simulink model "tqdtqr_rebuild_V3"  (R2021b)
settings: Solver=VariableStepAuto  StartTime=0.0  StopTime=10.0  RelTol=1e-3
undefined symbols (not defined in the file): ATQD_AfterTqMinGain_X_Deg, ATQD_APSCreepBaseTqD_X_kph, ATQD_APSCreepBaseTqD_Y_Deg, ATQD_APSCreepBaseTqR_X_kph, ATQD_APSCreepBaseTqR_Y_Deg, ATQD_APSCreepIterm_X_kph, ATQD_APSCreepIterm_Y_kph, ATQD_APSCreepPterm_X_kph, ATQD_APSCreepPterm_Y_kph, ATQD_APSDecReq_X_kph, ATQD_APSDecReq_Y_mps2, ATQD_APSDecReqCMD_X_kph, ATQD_APSDecReqTs_X_pct, ATQD_APSDecTimeGain_X_Deg, ATQD_APSDecTimeGain_Y_s, ATQD_APSReqLowSpd_X_Deg, ATQD_AutoHoldReleaseBPS_X_Deg, ATQD_AWDLoadTrqnsGain_X_kg, ATQD_AWDLoadTrqnsGain_Y_pct, ATQD_BOSEnBPSPosn_X_kph, ATQD_BOSMap_X_rpm, ATQD_BOSMap_Y_pct, ATQD_CreepBaseTqD_X_kph, ATQD_CreepBaseTqD_Y_Deg, ATQD_CreepBaseTqR_X_kph, ATQD_CreepBaseTqR_Y_Deg, ATQD_CreepBPSDisPosn_X_Deg, ATQD_CreepBPSDisPosnR_X_Deg, ATQD_CreepBPSEnPosn_X_Deg, ATQD_CreepBPSEnPosnR_X_Deg, ATQD_CreepDeltaTq_X_kph, ATQD_CreepIterm_X_kph, ATQD_CreepIterm_Y_kph, ATQD_CreepItermMaxLimit_X_pct, ATQD_CreepPreloadTime_X_kph, ATQD_CreepPreloadTq_X_kph, ATQD_CreepPreloadTq_Y_s, ATQD_CreepProtTq_X_Deg, ATQD_CreepPterm_X_kph, ATQD_CreepPterm_Y_kph, ATQD_CreepRrTqSpRat_X_rpm, ATQD_CreepRrTqSpRat_Y_Nm, ATQD_CreepTargetSpdD_X_pct, ATQD_CreepTargetSpdR_X_pct, ATQD_CreepUpLimitTq_X_rpm, ATQD_DecIneOPDHoldEnDelay_X_Deg, ATQD_DecIneOPDHoldEnDelay_Y_bar, ATQD_ECOTqMapD_X_rpm, ATQD_ECOTqMapD_Y_pct, ATQD_EMTqMapD_X_rpm, ATQD_EMTqMapD_Y_pct, ATQD_EOPDTqMapDCon_X_rpm, ATQD_EOPDTqMapDCon_Y_Deg, ATQD_EstInitVehWeight_X_c, ATQD_FAfterTqCMDGain_X_rpm, ATQD_FAfterTqCMDGain_Y_pct, ATQD_ForceLowSpd_X_Deg, ATQD_ForcePLimitSpd_X_Deg, ATQD_FrLossMAPLowV_X_rpm, ATQD_FrLossMAPLowV_Y_Nm ... (+949)
libraries: simulink x235, hcu_lib x208, tqr x63, tqd x6
(part 8 of 37)

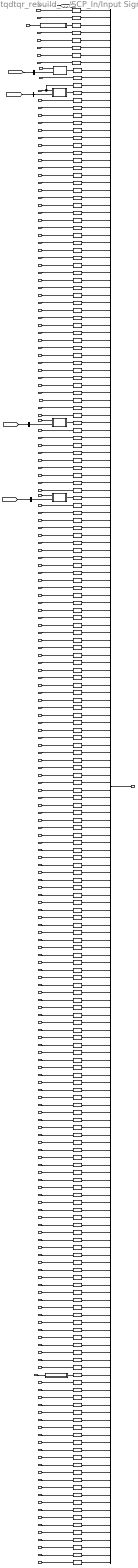
== system tqdtqr_rebuild_V3/SCP_In/Input Signal ==
  BInInvalid_outputs : Inport
  task_time_s : Inport  Port=2
  VDHP_ActAPSPosn_pct : Inport  Port=3
  VDHP_LowIdleAccPedal_flg : Inport  Port=4
  VPMM_PowerSta_enum : Inport  Port=5
  VPMM_DrivetrainSelect_enum : Inport  Port=6
  VPMM_SysPowerMode_enum : Inport  Port=7
  VPMM_DrSeatSta_enum : Inport  Port=8
  VINP_VehSpeed_kph : Inport  Port=9
  VINP_BrkSwSta_flg : Inport  Port=10
  VINP_BrkSwV_flg : Inport  Port=11
  VINP_BrkPedalPos_pct : Inport  Port=12
  VINP_BrkPedalPosSta_flg : Inport  Port=13
  VINP_FrPTCSActive_flg : Inport  Port=14
  VINP_RrPTCSActive_flg : Inport  Port=15
  VINP_FrntAxlTrqReqDrv_Nm : Inport  Port=16
  VINP_RearAxlTrqReqDrv_Nm : Inport  Port=17
  VINP_FrRBCActive_flg : Inport  Port=18
  VINP_RrRBCActive_flg : Inport  Port=19
  VINP_FrntAxlTrqReqBrk_Nm : Inport  Port=20
  VINP_RearAxlTrqReqBrk_Nm : Inport  Port=21
  VINP_CrashOutputSts_enum : Inport  Port=22
  VINP_LongAccel_Gps : Inport  Port=23
  VINP_EPBCarWashMode_flg : Inport  Port=24
  VINP_EPBErrSta_enum : Inport  Port=25
  VINP_EPBSta_enum : Inport  Port=26
  VINP_DOASta_flg : Inport  Port=27
  VINP_GRADE_Deg : Inport  Port=28
  VINP_HSAActive_flg : Inport  Port=29
  VINP_DriverSeatBeltCmd_flg : Inport  Port=30
  VINP_AVHActive_flg : Inport  Port=31
  VINP_PsngrSeatBeltCmd_flg : Inport  Port=32
  VINP_RDriverSeatBeltCmd_flg : Inport  Port=33
  VINP_RCenterSeatBeltCmd_flg : Inport  Port=34
  VINP_RPsngrSeatBeltCmd_flg : Inport  Port=35
  VINP_YawRate_degps : Inport  Port=36
  VINP_SASAngle_Deg : Inport  Port=37
  VINP_ESCActive_flg : Inport  Port=38
  VINP_ABSActive_flg : Inport  Port=39
  VINP_LFRawWhlSpeed_kph : Inport  Port=40
  VINP_LRRawWhlSpeed_kph : Inport  Port=41
  VINP_RFRawWhlSpeed_kph : Inport  Port=42
  VINP_RRRawWhlSpeed_kph : Inport  Port=43
  VINP_ESCOFFStatus_enum : Inport  Port=44
  VINP_MCPressure_bar : Inport  Port=45
  VINP_IVIPWModeReq_enum : Inport  Port=46
  VINP_IVICreepSWReq_flg : Inport  Port=47
  VINP_RollModeSWCmd_enum : Inport  Port=48
  VINP_IVIPwrLockSW_enum : Inport  Port=49
  VINP_IVIISAOffsetSpd_enum : Inport  Port=50
  VINP_Distanceunit_flg : Inport  Port=51
  VINP_SmartEcoModeSW_flg : Inport  Port=52
  VINP_IVISnowModeCmd_flg : Inport  Port=53
  VINP_IVIACCAdaptiveSta_flg : Inport  Port=54
  VINP_IVITrailerModeSWSta_flg : Inport  Port=55
  VINP_ShifterHandleCmd_enum : Inport  Port=56
  VINP_HVBPwrAvailDchrg_kW : Inport  Port=57
  VINP_HVBPwrAvailChrg_kW : Inport  Port=58
  VINP_HVBattErr_flg : Inport  Port=59
  VINP_DCDCFaultSta_enum : Inport  Port=60
  VINP_ChrgPlugSta_enum : Inport  Port=61
  VINP_HVBattSOC_pct : Inport  Port=62
  VINP_HVBattSOCDis_pct : Inport  Port=63
  VINP_HVBMTempMax_C : Inport  Port=64
  VINP_HVBMTempMin_C : Inport  Port=65
  VINP_ShifterFailsta_enum : Inport  Port=66
  VINP_CANMsgValidMCUNR1_flg : Inport  Port=67
  VINP_FrEDURotateDirctionNidec_enum : Inport  Port=68
  VINP_FrEDURotateDirction_enum : Inport  Port=69
  VINP_RrEDURotateDirctionNidec_enum : Inport  Port=70
  VINP_RrEDURotateDirction_enum : Inport  Port=71
  VINP_FrTMSpdNidec_rpm : Inport  Port=72
  VINP_FrTMSpd_rpm : Inport  Port=73
  VINP_RrTMSpdNidec_rpm : Inport  Port=74
  VINP_RrTMSpd_rpm : Inport  Port=75
  VINP_FrRegenAvailTqNidec_Nm : Inport  Port=76
  VINP_FrRegenAvailTq_Nm : Inport  Port=77
  VINP_RrRegenAvailTqNidec_Nm : Inport  Port=78
  VINP_RrRegenAvailTq_Nm : Inport  Port=79
  VINP_FrEDURealTMTqNidec_Nm : Inport  Port=80
  VINP_FrEDURealTMTq_Nm : Inport  Port=81
  VINP_RrEDURealTMTqNidec_Nm : Inport  Port=82
  VINP_RrEDURealTMTq_Nm : Inport  Port=83
  VINP_FrMotorAvailTqNidec_Nm : Inport  Port=84
  VINP_FrMotorAvailTq_Nm : Inport  Port=85
  VINP_RrMotorAvailTqNidec_Nm : Inport  Port=86
  VINP_RrMotorAvailTq_Nm : Inport  Port=87
  VINP_MCUWarnFNidec_enum : Inport  Port=88
  VINP_MCUWarnF_enum : Inport  Port=89
  VINP_MCUWarnRNidec_enum : Inport  Port=90
  VINP_MCUWarnR_enum : Inport  Port=91
  VINP_FrMCUDCBusVoltNidec_V : Inport  Port=92
  VINP_FrMCUDCBusVolt_V : Inport  Port=93
  VINP_RrMCUDCBusVoltNidec_V : Inport  Port=94
  VINP_RrMCUDCBusVolt_V : Inport  Port=95
  VINP_FrMCUTempNidec_C : Inport  Port=96
  VINP_FrMCUTemp_C : Inport  Port=97
  VINP_FrTMTempNidec_C : Inport  Port=98
  VINP_FrTMTemp_C : Inport  Port=99
  VINP_RrMCUTempNidec_C : Inport  Port=100
  VINP_RrMCUTemp_C : Inport  Port=101
  VINP_RrTMTempNidec_C : Inport  Port=102
  VINP_RrTMTemp_C : Inport  Port=103
  VINP_SWCResUpSta_flg : Inport  Port=104
  VINP_SWCSetdownSta_flg : Inport  Port=105
  VINP_SWCACCSta_flg : Inport  Port=106
  VINP_SWCCANCELSta_flg : Inport  Port=107
  VINP_SWC2LScrollUpSta_flg : Inport  Port=108
  VINP_SWC2LScrollDownSta_flg : Inport  Port=109
  VINP_SWC2LScrollPressSta_flg : Inport  Port=110
  VINP_SWC2LADASSta_flg : Inport  Port=111
  VINP_SWC2RScrollPressSta_flg : Inport  Port=112
  VINP_SWC2RScrollUpSta_flg : Inport  Port=113
  VINP_SWC2RScrollDownSta_flg : Inport  Port=114
  VINP_SWC2LDriveModeSta_flg : Inport  Port=115
  VINP_SWC2RRightSta_flg : Inport  Port=116
  VINP_SWC2RLeftSta_flg : Inport  Port=117
  VINP_SWCRegenUp_flg : Inport  Port=118
  VINP_SWC2RCustomizeSta_flg : Inport  Port=119
  VINP_SWC2LRegenUpSta_flg : Inport  Port=120
  VINP_SWC2RRegenDownSta_flg : Inport  Port=121
  VINP_SWCRegenDown_flg : Inport  Port=122
  VVMC_ADASForceIdle_flg : Inport  Port=123
  VVMC_ACCRequiredAccel_mps2 : Inport  Port=124
  VVMC_ACCVehHoldReq_flg : Inport  Port=125
  VVMC_ADASActive_flg : Inport  Port=126
  VVMC_ADASWhlTqReq_Nm : Inport  Port=127
  VVMC_CruzActive_flg : Inport  Port=128
  VVMC_CruzWhlTqReq_Nm : Inport  Port=129
  VVMC_MSAActive_flg : Inport  Port=130
  VVMC_MSAWhlTqReq_Nm : Inport  Port=131
  VVMC_APSActive_flg : Inport  Port=132
  VVMC_APSSpeedCMD_kph : Inport  Port=133
  VVMC_APSShiftPosnReq_enum : Inport  Port=134
  VVMC_ACCPedalOvrd_flg : Inport  Port=135
  VVMC_LongAcc_Gps : Inport  Port=136
  VVMC_ActMaxSlideRate_pct : Inport  Port=137
  VVMC_EstSlope_Deg : Inport  Port=138
  VVMC_APSReq_enum : Inport  Port=139
  VVMC_RWDRDCActive_enum : Inport  Port=140
  VVMC_ActLRSlideRate_pct : Inport  Port=141
  VVMC_ActRRSlideRate_pct : Inport  Port=142
  VVMC_ActStESCYaw_Dps : Inport  Port=143
  VVMC_CCCtrlSta_enum : Inport  Port=144
  VVMC_MSACtrlSta_enum : Inport  Port=145
  VVMC_LVDAACCStatusInformation_flg : Inport  Port=146
  VVMC_ACCObjDist_m : Inport  Port=147
  VVMC_MeterIndSpeed_raw32 : Inport  Port=148
  VVMC_RearTqRatio_rat : Inport  Port=149
  VVMC_CalibratedGyroY_Dps : Inport  Port=150
  VVMC_CAASActive_flg : Inport  Port=151
  VVMC_SetACCDisableAPS_flg : Inport  Port=152
  VVMC_CCPedalOvrd_flg : Inport  Port=153
  VVMC_MSAWhlTqActive_flg : Inport  Port=154
  VINP_BrakeSWGPIO_flg : Inport  Port=155
  VINP_CrashSignalGPIO_flg : Inport  Port=156
  VINP_DrDoorSW_flg : Inport  Port=157
  VINP_SeatSW_flg : Inport  Port=158
  VINP_HoodSW_flg : Inport  Port=159
  VINP_TailgateSW_flg : Inport  Port=160
  VINP_PsDoorSW_flg : Inport  Port=161
  VINP_RRDoorSW_flg : Inport  Port=162
  VINP_RLDoorSW_flg : Inport  Port=163
  VBCM_BrakeLamp_flg : Inport  Port=164
  VBCM_UserNow_enum : Inport  Port=165
  VINP_ADASISASta_enum : Inport  Port=166
  VINP_ADASVehSpdLim_enum : Inport  Port=167
  VINP_ADASACCSta_enum : Inport  Port=168
  VINP_ADASSLIFSpdLim_enum : Inport  Port=169
  VINP_ADASAEBSta_enum : Inport  Port=170
  VINP_ACCVehHoldReq_flg : Inport  Port=171
  VINP_FlashRegenMode_enum : Inport  Port=172
  VINP_VehicleType_enum : Inport  Port=173
  VINP_SWCType_enum : Inport  Port=174
  VINP_CAASSta_enum : Inport  Port=175
  VINP_APSStaSystem_enum : Inport  Port=176
  VDDM_VCURAPSErrLv2_flg : Inport  Port=177
  VDDM_VCURAPSErrLv3_flg : Inport  Port=178
  VDDM_EPBSigErrCFS_flg : Inport  Port=179
  VDDM_EPB1Err_flg : Inport  Port=180
  VDDM_ESC1Err_flg : Inport  Port=181
  VDDM_ESC5Err_flg : Inport  Port=182
  VDDM_LimpHomeAct_flg : Inport  Port=183
  VDDM_VehMalfunLevel_enum : Inport  Port=184
  VDDM_Shifter1Err_flg : Inport  Port=185
  VDDM_ShifterSigErrCFS_flg : Inport  Port=186
  VDDM_MCUF1Err_flg : Inport  Port=187
  VDDM_MCUR1Err_flg : Inport  Port=188
  VDDM_RegenErrCFS_flg : Inport  Port=189
  VDDM_4D2CErr_flg : Inport  Port=190
  VINP_PBWMotorPos_enum : Inport  Port=191
  VBCM_RegenModeUserSetting_enum : Inport  Port=192
  VINP_IVIEscapeModeCmd_flg : Inport  Port=193
  VINP_DIDExhibitMode_enum : Inport  Port=194
  VINP_DIDGetDynoMode_flg : Inport  Port=195
  VINP_CAN1BusOff_flg : Inport  Port=196
  VINP_CAN1BusError_flg : Inport  Port=197
  VINP_CAN2BusOff_flg : Inport  Port=198
  VINP_CAN2BusError_flg : Inport  Port=199
  VINP_DIDNVHPedalLim_flg : Inport  Port=200
  VINP_SCPSystemMode_enum : Inport  Port=201
  VDDM_EPB1NoComCFS_flg : Inport  Port=202
  VDDM_EPB1RCErrCFS_flg : Inport  Port=203
  VDDM_EPB1CSErrCFS_flg : Inport  Port=204
  VBCM_CTDCtrl_enum : Inport  Port=205
  VINP_FlashCrashDetd_flg : Inport  Port=206
  VINP_FlashCrashUnlockReq_flg : Inport  Port=207
  VBCM_CrashUnlkSuccess_flg : Inport  Port=208
  BrkPedalPos : Subsystem
  BrkSwSta : Subsystem
  Bus Creator : BusCreator  Inputs=208
  Bus Selector1 : BusSelector  OutputSignals=VTQD_ShifterHandleCmdInV_flg
  Bus Selector2 : BusSelector  OutputSignals=VTQD_ShifterFailstaInV_flg
  Bus Selector3 : BusSelector  OutputSignals=VINP_BrkSwStaSWInV_flg
  Bus Selector4 : BusSelector  OutputSignals=VINP_BrkPedalPosStaInV_flg
  Data Type Conversion{,1,6,9,13..14,17..18,20,25,33..34,37..40,53..54,58..61,68..83,88..99,120,123,125,127,129,132..134,137..139,143..146,191,203} (67 alike) : DataTypeConversion  OutDataTypeStr=single
  Data Type Conversion{2,7..8,10..12,15..16,21,24,26..32,35..36,43,47..51,55,63,100..119,121..122,124,126,128,131,142,147..158,170..176,178..183,185..190,192..196,199..201,205..207} (96 alike) : DataTypeConversion  OutDataTypeStr=boolean
  Data Type Conversion{3..5,19,22..23,41..42,44..46,52,56..57,62,64..67,84..87,130,135..136,140..141,159..169,177,184,197..198,202,204} (45 alike) : DataTypeConversion  OutDataTypeStr=uint8
  ShifterFailsta : Subsystem
  ShifterHandleCmd : Subsystem
  VDDM_LimpHomeAct_flg_ovrd : Subsystem
  VDHP_LowIdleAccPedal_flg_ovrd : Subsystem
  BSCPIn_outputs : Outport
  wires:
  Data Type Conversion177/1 -> Bus Creator/184  "VDDM_VehMalfunLevel_enum"
  Data Type Conversion184/1 -> Bus Creator/191  "VINP_PBWMotorPos_enum"
  VINP_EPBCarWashMode_flg/1 -> Data Type Conversion21/1
  Data Type Conversion107/1 -> Bus Creator/111  "VINP_SWC2LADASSta_flg"
  Data Type Conversion45/1 -> Bus Creator/49  "VINP_IVIPwrLockSW_enum"
  Data Type Conversion173/1 -> Bus Creator/180  "VDDM_EPB1Err_flg"
  VINP_RrMCUTemp_C/1 -> Data Type Conversion97/1
  VINP_ADASSLIFSpdLim_enum/1 -> Data Type Conversion163/1
  Data Type Conversion172/1 -> Bus Creator/179  "VDDM_EPBSigErrCFS_flg"
  Data Type Conversion179/1 -> Bus Creator/186  "VDDM_ShifterSigErrCFS_flg"
  Data Type Conversion148/1 -> Bus Creator/152  "VVMC_SetACCDisableAPS_flg"
  Data Type Conversion134/1 -> Bus Creator/138  "VVMC_EstSlope_Deg"
  Data Type Conversion108/1 -> Bus Creator/112  "VINP_SWC2RScrollPressSta_flg"
  Data Type Conversion127/1 -> Bus Creator/131  "VVMC_MSAWhlTqReq_Nm"
  VINP_CrashSignalGPIO_flg/1 -> Data Type Conversion150/1
  VINP_IVISnowModeCmd_flg/1 -> Data Type Conversion49/1
  VINP_IVIEscapeModeCmd_flg/1 -> Data Type Conversion186/1
  Data Type Conversion139/1 -> Bus Creator/143  "VVMC_ActStESCYaw_Dps"
  Data Type Conversion105/1 -> Bus Creator/109  "VINP_SWC2LScrollDownSta_flg"
  Data Type Conversion47/1 -> Bus Creator/51  "VINP_Distanceunit_flg"
  Data Type Conversion118/1 -> Bus Creator/122  "VINP_SWCRegenDown_flg"
  VINP_DCDCFaultSta_enum/1 -> Data Type Conversion56/1
  VINP_ADASISASta_enum/1 -> Data Type Conversion160/1
  VDDM_Shifter1Err_flg/1 -> Data Type Conversion178/1
  Data Type Conversion71/1 -> Bus Creator/75  "VINP_RrTMSpd_rpm"
  Data Type Conversion175/1 -> Bus Creator/182  "VDDM_ESC5Err_flg"
  Data Type Conversion171/1 -> Bus Creator/178  "VDDM_VCURAPSErrLv3_flg"
  Data Type Conversion32/1 -> Bus Creator/35  "VINP_RPsngrSeatBeltCmd_flg"
  Data Type Conversion140/1 -> Bus Creator/144  "VVMC_CCCtrlSta_enum"
  Data Type Conversion/1 -> Bus Creator/1  "task_time_s"
  Data Type Conversion131/1 -> Bus Creator/135  "VVMC_ACCPedalOvrd_flg"
  VINP_RrEDURealTMTqNidec_Nm/1 -> Data Type Conversion78/1
  Data Type Conversion89/1 -> Bus Creator/93  "VINP_FrMCUDCBusVolt_V"
  VDDM_ShifterSigErrCFS_flg/1 -> Data Type Conversion179/1
  Data Type Conversion126/1 -> Bus Creator/130  "VVMC_MSAActive_flg"
  VINP_RPsngrSeatBeltCmd_flg/1 -> Data Type Conversion32/1
  Data Type Conversion24/1 -> Bus Creator/27  "VINP_DOASta_flg"
  VINP_SWC2LScrollDownSta_flg/1 -> Data Type Conversion105/1
  Data Type Conversion174/1 -> Bus Creator/181  "VDDM_ESC1Err_flg"
  VDDM_EPB1Err_flg/1 -> Data Type Conversion173/1
  VINP_CAASSta_enum/1 -> Data Type Conversion168/1
  Data Type Conversion38/1 -> Bus Creator/41  "VINP_LRRawWhlSpeed_kph"
  Data Type Conversion75/1 -> Bus Creator/79  "VINP_RrRegenAvailTq_Nm"
  VVMC_ActLRSlideRate_pct/1 -> Data Type Conversion137/1
  VINP_RDriverSeatBeltCmd_flg/1 -> Data Type Conversion30/1
  Data Type Conversion116/1 -> Bus Creator/120  "VINP_SWC2LRegenUpSta_flg"
  Data Type Conversion11/1 -> Bus Creator/14  "VINP_FrPTCSActive_flg"
  VINP_ADASAEBSta_enum/1 -> Data Type Conversion164/1
  Data Type Conversion176/1 -> Bus Creator/183  "VTQD_LimpHomeAct_flg"
  VVMC_ActRRSlideRate_pct/1 -> Data Type Conversion138/1
  Data Type Conversion94/1 -> Bus Creator/98  "VINP_FrTMTempNidec_C"
  Data Type Conversion178/1 -> Bus Creator/185  "VDDM_Shifter1Err_flg"
  Data Type Conversion121/1 -> Bus Creator/125  "VVMC_ACCVehHoldReq_flg"
  Data Type Conversion138/1 -> Bus Creator/142  "VVMC_ActRRSlideRate_pct"
  VDDM_MCUR1Err_flg/1 -> Data Type Conversion181/1
  Data Type Conversion76/1 -> Bus Creator/80  "VINP_FrEDURealTMTqNidec_Nm"
  Data Type Conversion182/1 -> Bus Creator/189  "VDDM_RegenErrCFS_flg"
  Data Type Conversion103/1 -> Bus Creator/107  "VINP_SWCCANCELSta_flg"
  Data Type Conversion183/1 -> Bus Creator/190  "VDDM_4D2CErr_flg"
  Data Type Conversion157/1 -> Bus Creator/163  "VINP_RLDoorSW_flg"
  Data Type Conversion98/1 -> Bus Creator/102  "VINP_RrTMTempNidec_C"
  Data Type Conversion185/1 -> Bus Creator/192  "VBCM_RegenModeUserSetting_enum"
  VVMC_SetACCDisableAPS_flg/1 -> Data Type Conversion148/1
  VINP_LFRawWhlSpeed_kph/1 -> Data Type Conversion37/1
  Data Type Conversion21/1 -> Bus Creator/24  "VINP_EPBCarWashMode_flg"
  Data Type Conversion99/1 -> Bus Creator/103  "VINP_RrTMTemp_C"
  VINP_HVBMTempMin_C/1 -> Data Type Conversion61/1
  Data Type Conversion119/1 -> Bus Creator/123  "VVMC_ADASForceIdle_flg"
  Data Type Conversion18/1 -> Bus Creator/21  "VINP_RearAxlTrqReqBrk_Nm"
  VVMC_RearTqRatio_rat/1 -> Data Type Conversion145/1
  Data Type Conversion50/1 -> Bus Creator/54  "VINP_IVIACCAdaptiveSta_flg"
  Data Type Conversion55/1 -> Bus Creator/59  "VINP_HVBattErr_flg"
  VINP_DriverSeatBeltCmd_flg/1 -> Data Type Conversion27/1
  VINP_HVBPwrAvailChrg_kW/1 -> Data Type Conversion54/1
  VVMC_ActStESCYaw_Dps/1 -> Data Type Conversion139/1
  Data Type Conversion129/1 -> Bus Creator/133  "VVMC_APSSpeedCMD_kph"
  VINP_ESCActive_flg/1 -> Data Type Conversion35/1
  Data Type Conversion180/1 -> Bus Creator/187  "VDDM_MCUF1Err_flg"
  Data Type Conversion104/1 -> Bus Creator/108  "VINP_SWC2LScrollUpSta_flg"
  Bus Creator/1 -> BSCPIn_outputs/1  "BSCPIn_outputs"
  Data Type Conversion73/1 -> Bus Creator/77  "VINP_FrRegenAvailTq_Nm"
  Data Type Conversion4/1 -> Bus Creator/5  "VPMM_DrivetrainSelect_enum"
  Data Type Conversion97/1 -> Bus Creator/101  "VINP_RrMCUTemp_C"
  Data Type Conversion26/1 -> Bus Creator/29  "VINP_HSAActive_flg"
  Data Type Conversion181/1 -> Bus Creator/188  "VDDM_MCUR1Err_flg"
  Data Type Conversion46/1 -> Bus Creator/50  "VINP_IVIISAOffsetSpd_enum"
  Data Type Conversion186/1 -> Bus Creator/193  "VINP_IVIEscapeModeCmd_flg"
  Data Type Conversion113/1 -> Bus Creator/117  "VINP_SWC2RLeftSta_flg"
  Data Type Conversion96/1 -> Bus Creator/100  "VINP_RrMCUTempNidec_C"
  Data Type Conversion60/1 -> Bus Creator/64  "VINP_HVBMTempMax_C"
  VINP_FrntAxlTrqReqBrk_Nm/1 -> Data Type Conversion17/1
  Data Type Conversion90/1 -> Bus Creator/94  "VINP_RrMCUDCBusVoltNidec_V"
  VINP_FrMotorAvailTq_Nm/1 -> Data Type Conversion81/1
  Data Type Conversion15/1 -> Bus Creator/18  "VINP_FrRBCActive_flg"
  VINP_RRDoorSW_flg/1 -> Data Type Conversion156/1
  Data Type Conversion28/1 -> Bus Creator/31  "VINP_AVHActive_flg"
  Data Type Conversion92/1 -> Bus Creator/96  "VINP_FrMCUTempNidec_C"
  Data Type Conversion93/1 -> Bus Creator/97  "VINP_FrMCUTemp_C"
  VDDM_EPBSigErrCFS_flg/1 -> Data Type Conversion172/1
  Data Type Conversion10/1 -> Bus Creator/13  "VINP_BrkPedalPosSta_flg"
  Data Type Conversion114/1 -> Bus Creator/118  "VINP_SWCRegenUp_flg"
  Data Type Conversion91/1 -> Bus Creator/95  "VINP_RrMCUDCBusVolt_V"
  Data Type Conversion123/1 -> Bus Creator/127  "VVMC_ADASWhlTqReq_Nm"
  VVMC_CAASActive_flg/1 -> Data Type Conversion147/1
  Data Type Conversion95/1 -> Bus Creator/99  "VINP_FrTMTemp_C"
  Data Type Conversion100/1 -> Bus Creator/104  "VINP_SWCResUpSta_flg"
  Data Type Conversion56/1 -> Bus Creator/60  "VINP_DCDCFaultSta_enum"
  Data Type Conversion101/1 -> Bus Creator/105  "VINP_SWCSetdownSta_flg"
  VINP_IVITrailerModeSWSta_flg/1 -> Data Type Conversion51/1
  Data Type Conversion63/1 -> Bus Creator/67  "VINP_CANMsgValidMCUNR1_flg"
  VINP_SWCRegenDown_flg/1 -> Data Type Conversion118/1
  VINP_RrRegenAvailTq_Nm/1 -> Data Type Conversion75/1
  VINP_RrMCUDCBusVolt_V/1 -> Data Type Conversion91/1
  Data Type Conversion133/1 -> Bus Creator/137  "VVMC_ActMaxSlideRate_pct"
  Data Type Conversion102/1 -> Bus Creator/106  "VINP_SWCACCSta_flg"
  VINP_RrMCUTempNidec_C/1 -> Data Type Conversion96/1
  Data Type Conversion80/1 -> Bus Creator/84  "VINP_FrMotorAvailTqNidec_Nm"
  VINP_SWC2LADASSta_flg/1 -> Data Type Conversion107/1
  Data Type Conversion106/1 -> Bus Creator/110  "VINP_SWC2LScrollPressSta_flg"
  VINP_SWCACCSta_flg/1 -> Data Type Conversion102/1
  Data Type Conversion130/1 -> Bus Creator/134  "VVMC_APSShiftPosnReq_enum"
  Data Type Conversion110/1 -> Bus Creator/114  "VINP_SWC2RScrollDownSta_flg"
  VINP_FrMCUTemp_C/1 -> Data Type Conversion93/1
  Data Type Conversion111/1 -> Bus Creator/115  "VINP_SWC2LDriveModeSta_flg"
  Data Type Conversion117/1 -> Bus Creator/121  "VINP_SWC2RRegenDownSta_flg"
  Data Type Conversion112/1 -> Bus Creator/116  "VINP_SWC2RRightSta_flg"
  VINP_AVHActive_flg/1 -> Data Type Conversion28/1
  VINP_SmartEcoModeSW_flg/1 -> Data Type Conversion48/1
  Data Type Conversion39/1 -> Bus Creator/42  "VINP_RFRawWhlSpeed_kph"
  VINP_RRRawWhlSpeed_kph/1 -> Data Type Conversion40/1
  VPMM_PowerSta_enum/1 -> Data Type Conversion3/1
  Data Type Conversion37/1 -> Bus Creator/40  "VINP_LFRawWhlSpeed_kph"
  Data Type Conversion109/1 -> Bus Creator/113  "VINP_SWC2RScrollUpSta_flg"
  VVMC_ActMaxSlideRate_pct/1 -> Data Type Conversion133/1
  Data Type Conversion115/1 -> Bus Creator/119  "VINP_SWC2RCustomizeSta_flg"
  Data Type Conversion137/1 -> Bus Creator/141  "VVMC_ActLRSlideRate_pct"
  Data Type Conversion149/1 -> Bus Creator/155  "VINP_BrakeSWGPIO_flg"
  VVMC_CalibratedGyroY_Dps/1 -> Data Type Conversion146/1
  Data Type Conversion120/1 -> Bus Creator/124  "VVMC_ACCRequiredAccel_mps2"
  VVMC_ADASWhlTqReq_Nm/1 -> Data Type Conversion123/1
  VVMC_ADASForceIdle_flg/1 -> Data Type Conversion119/1
  VINP_DrDoorSW_flg/1 -> Data Type Conversion151/1
  Data Type Conversion122/1 -> Bus Creator/126  "VVMC_ADASActive_flg"
  Data Type Conversion125/1 -> Bus Creator/129  "VVMC_CruzWhlTqReq_Nm"
  Data Type Conversion124/1 -> Bus Creator/128  "VVMC_CruzActive_flg"
  Data Type Conversion84/1 -> Bus Creator/88  "VINP_MCUWarnFNidec_enum"
  Data Type Conversion132/1 -> Bus Creator/136  "VVMC_LongAcc_Gps"
  Data Type Conversion142/1 -> Bus Creator/146  "VVMC_LVDAACCStatusInformation_flg"
  Data Type Conversion128/1 -> Bus Creator/132  "VVMC_APSActive_flg"
  VVMC_MSAWhlTqReq_Nm/1 -> Data Type Conversion127/1
  VINP_SASAngle_Deg/1 -> Data Type Conversion34/1
  VINP_RrTMSpd_rpm/1 -> Data Type Conversion71/1
  Data Type Conversion135/1 -> Bus Creator/139  "VVMC_APSReq_enum"
  Data Type Conversion2/1 -> Bus Creator/3  "VTQD_LowIdleAccPedal_flg"
  Data Type Conversion27/1 -> Bus Creator/30  "VINP_DriverSeatBeltCmd_flg"
  Data Type Conversion14/1 -> Bus Creator/17  "VINP_RearAxlTrqReqDrv_Nm"
  Data Type Conversion136/1 -> Bus Creator/140  "VTQD_RDCActive_enum"
  Data Type Conversion141/1 -> Bus Creator/145  "VVMC_MSACtrlSta_enum"
  VDDM_VehMalfunLevel_enum/1 -> Data Type Conversion177/1
  Data Type Conversion143/1 -> Bus Creator/147  "VVMC_ACCObjDist_m"
  Data Type Conversion144/1 -> Bus Creator/148  "VVMC_MeterIndSpeed_raw32"
  Data Type Conversion145/1 -> Bus Creator/149  "VVMC_RearTqRatio_rat"
  VINP_SWCRegenUp_flg/1 -> Data Type Conversion114/1
  VINP_FrEDURealTMTqNidec_Nm/1 -> Data Type Conversion76/1
  VINP_RrRegenAvailTqNidec_Nm/1 -> Data Type Conversion74/1
  VINP_RrTMTemp_C/1 -> Data Type Conversion99/1
  Data Type Conversion151/1 -> Bus Creator/157  "VINP_DrDoorSW_flg"
  Data Type Conversion152/1 -> Bus Creator/158  "VINP_SeatSW_flg"
  Data Type Conversion146/1 -> Bus Creator/150  "VVMC_CalibratedGyroY_Dps"
  Data Type Conversion150/1 -> Bus Creator/156  "VINP_CrashSignalGPIO_flg"
  VINP_RearAxlTrqReqDrv_Nm/1 -> Data Type Conversion14/1
  Data Type Conversion147/1 -> Bus Creator/151  "VVMC_CAASActive_flg"
  VDDM_MCUF1Err_flg/1 -> Data Type Conversion180/1
  VINP_HSAActive_flg/1 -> Data Type Conversion26/1
  Data Type Conversion155/1 -> Bus Creator/161  "VINP_PsDoorSW_flg"
  Data Type Conversion158/1 -> Bus Creator/164  "VBCM_BrakeLamp_flg"
  Data Type Conversion153/1 -> Bus Creator/159  "VINP_HoodSW_flg"
  VINP_SWC2RScrollUpSta_flg/1 -> Data Type Conversion109/1
  VINP_RearAxlTrqReqBrk_Nm/1 -> Data Type Conversion18/1
  VINP_MCUWarnR_enum/1 -> Data Type Conversion87/1
  Data Type Conversion156/1 -> Bus Creator/162  "VINP_RRDoorSW_flg"
  Data Type Conversion59/1 -> Bus Creator/63  "VINP_HVBattSOCDis_pct"
  VVMC_APSReq_enum/1 -> Data Type Conversion135/1
  VINP_RLDoorSW_flg/1 -> Data Type Conversion157/1
  Data Type Conversion154/1 -> Bus Creator/160  "VINP_TailgateSW_flg"
  Data Type Conversion162/1 -> Bus Creator/168  "VINP_ADASACCSta_enum"
  Data Type Conversion161/1 -> Bus Creator/167  "VINP_ADASVehSpdLim_enum"
  Data Type Conversion159/1 -> Bus Creator/165  "VBCM_UserNow_enum"
  VINP_ADASACCSta_enum/1 -> Data Type Conversion162/1
  Data Type Conversion35/1 -> Bus Creator/38  "VINP_ESCActive_flg"
  Data Type Conversion164/1 -> Bus Creator/170  "VINP_ADASAEBSta_enum"
  VINP_PsngrSeatBeltCmd_flg/1 -> Data Type Conversion29/1
  Data Type Conversion163/1 -> Bus Creator/169  "VINP_ADASSLIFSpdLim_enum"
  VPMM_SysPowerMode_enum/1 -> Data Type Conversion5/1
  Data Type Conversion165/1 -> Bus Creator/172  "VINP_FlashRegenMode_enum"
  Data Type Conversion36/1 -> Bus Creator/39  "VINP_ABSActive_flg"
  Data Type Conversion160/1 -> Bus Creator/166  "VINP_ADASISASta_enum"
  VINP_FrMCUDCBusVolt_V/1 -> Data Type Conversion89/1
  VINP_RollModeSWCmd_enum/1 -> Data Type Conversion44/1
  Data Type Conversion166/1 -> Bus Creator/173  "VINP_VehicleType_enum"
  Data Type Conversion78/1 -> Bus Creator/82  "VINP_RrEDURealTMTqNidec_Nm"
  VINP_ESCOFFStatus_enum/1 -> Data Type Conversion41/1
  Data Type Conversion83/1 -> Bus Creator/87  "VINP_RrMotorAvailTq_Nm"
  Data Type Conversion167/1 -> Bus Creator/174  "VINP_SWCType_enum"
  Data Type Conversion169/1 -> Bus Creator/176  "VINP_APSStaSystem_enum"
  Data Type Conversion170/1 -> Bus Creator/177  "VDDM_VCURAPSErrLv2_flg"
  Data Type Conversion168/1 -> Bus Creator/175  "VINP_CAASSta_enum"
  Data Type Conversion1/1 -> Bus Creator/2  "VTQD_ActAPSPosn_pct"
  VINP_RrMCUDCBusVoltNidec_V/1 -> Data Type Conversion90/1
  Data Type Conversion6/1 -> Bus Creator/8  "VINP_VehSpeed_kph"
  Data Type Conversion43/1 -> Bus Creator/47  "VINP_IVICreepSWReq_flg"
  Data Type Conversion5/1 -> Bus Creator/6  "VPMM_SysPowerMode_enum"
  Data Type Conversion3/1 -> Bus Creator/4  "VPMM_PowerSta_enum"
  Data Type Conversion12/1 -> Bus Creator/15  "VINP_RrPTCSActive_flg"
  Data Type Conversion81/1 -> Bus Creator/85  "VINP_FrMotorAvailTq_Nm"
  Data Type Conversion19/1 -> Bus Creator/22  "VINP_CrashOutputSts_enum"
  Data Type Conversion9/1 -> Bus Creator/12  "VTQD_ActBPSPosn_pct"
  VINP_CANMsgValidMCUNR1_flg/1 -> Data Type Conversion63/1
  Data Type Conversion58/1 -> Bus Creator/62  "VINP_HVBattSOC_pct"
  VVMC_ADASActive_flg/1 -> Data Type Conversion122/1
  VINP_SWC2RScrollPressSta_flg/1 -> Data Type Conversion108/1
  Data Type Conversion13/1 -> Bus Creator/16  "VINP_FrntAxlTrqReqDrv_Nm"
  VINP_PBWMotorPos_enum/1 -> Data Type Conversion184/1
  Data Type Conversion16/1 -> Bus Creator/19  "VINP_RrRBCActive_flg"
  VBCM_RegenModeUserSetting_enum/1 -> Data Type Conversion185/1
  Data Type Conversion17/1 -> Bus Creator/20  "VINP_FrntAxlTrqReqBrk_Nm"
  VINP_SWC2RCustomizeSta_flg/1 -> Data Type Conversion115/1
  VINP_ChrgPlugSta_enum/1 -> Data Type Conversion57/1
  Data Type Conversion20/1 -> Bus Creator/23  "VINP_LongAccel_Gps"
  Data Type Conversion22/1 -> Bus Creator/25  "VINP_EPBErrSta_enum"
  Data Type Conversion25/1 -> Bus Creator/28  "VINP_GRADE_Deg"
  Data Type Conversion23/1 -> Bus Creator/26  "VINP_EPBSta_enum"
  VVMC_ACCObjDist_m/1 -> Data Type Conversion143/1
  VDHP_ActAPSPosn_pct/1 -> Data Type Conversion1/1
  VINP_TailgateSW_flg/1 -> Data Type Conversion154/1
  VINP_SWC2LDriveModeSta_flg/1 -> Data Type Conversion111/1
  Data Type Conversion85/1 -> Bus Creator/89  "VINP_MCUWarnF_enum"
  VVMC_APSActive_flg/1 -> Data Type Conversion128/1
  VINP_FrEDURotateDirctionNidec_enum/1 -> Data Type Conversion64/1
  VINP_SWC2RRegenDownSta_flg/1 -> Data Type Conversion117/1
  VINP_IVIPWModeReq_enum/1 -> Data Type Conversion42/1
  VINP_HVBattErr_flg/1 -> Data Type Conversion55/1
  VINP_SWC2RScrollDownSta_flg/1 -> Data Type Conversion110/1
  Data Type Conversion29/1 -> Bus Creator/32  "VINP_PsngrSeatBeltCmd_flg"
  Data Type Conversion88/1 -> Bus Creator/92  "VINP_FrMCUDCBusVoltNidec_V"
  VINP_FrPTCSActive_flg/1 -> Data Type Conversion11/1
  VINP_RrTMSpdNidec_rpm/1 -> Data Type Conversion70/1
  Data Type Conversion30/1 -> Bus Creator/33  "VINP_RDriverSeatBeltCmd_flg"
  VVMC_ACCRequiredAccel_mps2/1 -> Data Type Conversion120/1
  Data Type Conversion31/1 -> Bus Creator/34  "VINP_RCenterSeatBeltCmd_flg"
  Data Type Conversion34/1 -> Bus Creator/37  "VINP_SASAngle_Deg"
  Data Type Conversion33/1 -> Bus Creator/36  "VINP_YawRate_degps"
  Data Type Conversion42/1 -> Bus Creator/46  "VINP_IVIPWModeReq_enum"
  VDDM_VCURAPSErrLv2_flg/1 -> Data Type Conversion170/1
  Data Type Conversion44/1 -> Bus Creator/48  "VINP_RollModeSWCmd_enum"
  VINP_HVBattSOC_pct/1 -> Data Type Conversion58/1
  Data Type Conversion41/1 -> Bus Creator/44  "VINP_ESCOFFStatus_enum"
  Data Type Conversion40/1 -> Bus Creator/43  "VINP_RRRawWhlSpeed_kph"
  VINP_SWC2RRightSta_flg/1 -> Data Type Conversion112/1
  VINP_SWC2LScrollPressSta_flg/1 -> Data Type Conversion106/1
  VINP_RrMotorAvailTqNidec_Nm/1 -> Data Type Conversion82/1
  Data Type Conversion49/1 -> Bus Creator/53  "VINP_IVISnowModeCmd_flg"
  Data Type Conversion51/1 -> Bus Creator/55  "VINP_IVITrailerModeSWSta_flg"
  Data Type Conversion82/1 -> Bus Creator/86  "VINP_RrMotorAvailTqNidec_Nm"
  VINP_RrTMTempNidec_C/1 -> Data Type Conversion98/1
  Data Type Conversion72/1 -> Bus Creator/76  "VINP_FrRegenAvailTqNidec_Nm"
  VINP_RFRawWhlSpeed_kph/1 -> Data Type Conversion39/1
  VINP_SWC2LScrollUpSta_flg/1 -> Data Type Conversion104/1
  Data Type Conversion48/1 -> Bus Creator/52  "VINP_SmartEcoModeSW_flg"
  VBCM_BrakeLamp_flg/1 -> Data Type Conversion158/1
  VINP_FrTMTempNidec_C/1 -> Data Type Conversion94/1
  VINP_ABSActive_flg/1 -> Data Type Conversion36/1
  Data Type Conversion53/1 -> Bus Creator/57  "VINP_HVBPwrAvailDchrg_kW"
  Data Type Conversion54/1 -> Bus Creator/58  "VINP_HVBPwrAvailChrg_kW"
  Data Type Conversion79/1 -> Bus Creator/83  "VINP_RrEDURealTMTq_Nm"
  Data Type Conversion52/1 -> Bus Creator/56  "VTQD_ShifterHandleCmd_enum"
  Data Type Conversion69/1 -> Bus Creator/73  "VINP_FrTMSpd_rpm"
  Data Type Conversion57/1 -> Bus Creator/61  "VINP_ChrgPlugSta_enum"
  VDDM_ESC1Err_flg/1 -> Data Type Conversion174/1
  Data Type Conversion61/1 -> Bus Creator/65  "VINP_HVBMTempMin_C"
  Data Type Conversion62/1 -> Bus Creator/66  "VTQD_ShifterFailsta_enum"
  Data Type Conversion67/1 -> Bus Creator/71  "VINP_RrEDURotateDirction_enum"
  Data Type Conversion68/1 -> Bus Creator/72  "VINP_FrTMSpdNidec_rpm"
  Data Type Conversion65/1 -> Bus Creator/69  "VINP_FrEDURotateDirction_enum"
  Data Type Conversion66/1 -> Bus Creator/70  "VINP_RrEDURotateDirctionNidec_enum"
  VINP_RrPTCSActive_flg/1 -> Data Type Conversion12/1
  Data Type Conversion64/1 -> Bus Creator/68  "VINP_FrEDURotateDirctionNidec_enum"
  Data Type Conversion74/1 -> Bus Creator/78  "VINP_RrRegenAvailTqNidec_Nm"
  VINP_FrMCUDCBusVoltNidec_V/1 -> Data Type Conversion88/1
  Data Type Conversion70/1 -> Bus Creator/74  "VINP_RrTMSpdNidec_rpm"
  Data Type Conversion77/1 -> Bus Creator/81  "VINP_FrEDURealTMTq_Nm"
  Data Type Conversion87/1 -> Bus Creator/91  "VINP_MCUWarnR_enum"
  VINP_SWCResUpSta_flg/1 -> Data Type Conversion100/1
  VINP_HVBPwrAvailDchrg_kW/1 -> Data Type Conversion53/1
  VINP_RrEDURotateDirctionNidec_enum/1 -> Data Type Conversion66/1
  Data Type Conversion86/1 -> Bus Creator/90  "VINP_MCUWarnRNidec_enum"
  VINP_FrntAxlTrqReqDrv_Nm/1 -> Data Type Conversion13/1
  VINP_ADASVehSpdLim_enum/1 -> Data Type Conversion161/1
  VINP_RCenterSeatBeltCmd_flg/1 -> Data Type Conversion31/1
  VINP_IVICreepSWReq_flg/1 -> Data Type Conversion43/1
  VVMC_RWDRDCActive_enum/1 -> Data Type Conversion136/1
  VINP_BrakeSWGPIO_flg/1 -> Data Type Conversion149/1
  VDDM_ESC5Err_flg/1 -> Data Type Conversion175/1
  VINP_IVIISAOffsetSpd_enum/1 -> Data Type Conversion46/1
  VINP_FrTMTemp_C/1 -> Data Type Conversion95/1
  VVMC_LVDAACCStatusInformation_flg/1 -> Data Type Conversion142/1
  VINP_SWC2RLeftSta_flg/1 -> Data Type Conversion113/1
  VINP_RrEDURotateDirction_enum/1 -> Data Type Conversion67/1
  VVMC_CCCtrlSta_enum/1 -> Data Type Conversion140/1
  VVMC_MSACtrlSta_enum/1 -> Data Type Conversion141/1
  VVMC_MSAActive_flg/1 -> Data Type Conversion126/1
  VINP_LongAccel_Gps/1 -> Data Type Conversion20/1
  VINP_EPBErrSta_enum/1 -> Data Type Conversion22/1
  VINP_GRADE_Deg/1 -> Data Type Conversion25/1
  VVMC_EstSlope_Deg/1 -> Data Type Conversion134/1
  task_time_s/1 -> Data Type Conversion/1
  VVMC_MeterIndSpeed_raw32/1 -> Data Type Conversion144/1
  VINP_FrMotorAvailTqNidec_Nm/1 -> Data Type Conversion80/1
  VINP_SeatSW_flg/1 -> Data Type Conversion152/1
  VINP_RrRBCActive_flg/1 -> Data Type Conversion16/1
  VINP_PsDoorSW_flg/1 -> Data Type Conversion155/1
  VINP_DOASta_flg/1 -> Data Type Conversion24/1
  VINP_EPBSta_enum/1 -> Data Type Conversion23/1
  VVMC_ACCVehHoldReq_flg/1 -> Data Type Conversion121/1
  VINP_YawRate_degps/1 -> Data Type Conversion33/1
  VINP_VehSpeed_kph/1 -> Data Type Conversion6/1
  VINP_BrkPedalPosSta_flg/1 -> Data Type Conversion10/1
  VINP_SWC2LRegenUpSta_flg/1 -> Data Type Conversion116/1
  VINP_MCUWarnRNidec_enum/1 -> Data Type Conversion86/1
  VINP_LRRawWhlSpeed_kph/1 -> Data Type Conversion38/1
  VPMM_DrivetrainSelect_enum/1 -> Data Type Conversion4/1
  VINP_FrRBCActive_flg/1 -> Data Type Conversion15/1
  VINP_FrRegenAvailTq_Nm/1 -> Data Type Conversion73/1
  VINP_FrTMSpdNidec_rpm/1 -> Data Type Conversion68/1
  VINP_FrRegenAvailTqNidec_Nm/1 -> Data Type Conversion72/1
  VINP_FrMCUTempNidec_C/1 -> Data Type Conversion92/1
  VDDM_VCURAPSErrLv3_flg/1 -> Data Type Conversion171/1
  VINP_MCUWarnFNidec_enum/1 -> Data Type Conversion84/1
  VINP_IVIPwrLockSW_enum/1 -> Data Type Conversion45/1
  VINP_FlashRegenMode_enum/1 -> Data Type Conversion165/1
  VINP_Distanceunit_flg/1 -> Data Type Conversion47/1
  VINP_SWCType_enum/1 -> Data Type Conversion167/1
  VDDM_4D2CErr_flg/1 -> Data Type Conversion183/1
  VINP_CrashOutputSts_enum/1 -> Data Type Conversion19/1
  VINP_RrMotorAvailTq_Nm/1 -> Data Type Conversion83/1
  VINP_FrEDURotateDirction_enum/1 -> Data Type Conversion65/1
  VINP_IVIACCAdaptiveSta_flg/1 -> Data Type Conversion50/1
  VVMC_ACCPedalOvrd_flg/1 -> Data Type Conversion131/1
  VINP_APSStaSystem_enum/1 -> Data Type Conversion169/1
  VINP_VehicleType_enum/1 -> Data Type Conversion166/1
  VINP_HoodSW_flg/1 -> Data Type Conversion153/1
  VDDM_RegenErrCFS_flg/1 -> Data Type Conversion182/1
  VINP_HVBMTempMax_C/1 -> Data Type Conversion60/1
  VINP_RrEDURealTMTq_Nm/1 -> Data Type Conversion79/1
  VINP_FrEDURealTMTq_Nm/1 -> Data Type Conversion77/1
  VINP_MCUWarnF_enum/1 -> Data Type Conversion85/1
  VINP_SWCCANCELSta_flg/1 -> Data Type Conversion103/1
  VINP_SWCSetdownSta_flg/1 -> Data Type Conversion101/1
  VVMC_CruzWhlTqReq_Nm/1 -> Data Type Conversion125/1
  VVMC_LongAcc_Gps/1 -> Data Type Conversion132/1
  VVMC_APSSpeedCMD_kph/1 -> Data Type Conversion129/1
  VBCM_UserNow_enum/1 -> Data Type Conversion159/1
  VINP_FrTMSpd_rpm/1 -> Data Type Conversion69/1
  VVMC_APSShiftPosnReq_enum/1 -> Data Type Conversion130/1
  VINP_HVBattSOCDis_pct/1 -> Data Type Conversion59/1
  VVMC_CruzActive_flg/1 -> Data Type Conversion124/1
  VDDM_LimpHomeAct_flg/1 -> VDDM_LimpHomeAct_flg_ovrd/1(Signal_In)
  VDHP_LowIdleAccPedal_flg/1 -> VDHP_LowIdleAccPedal_flg_ovrd/1(Signal_In)
  VDHP_LowIdleAccPedal_flg_ovrd/1(Signal_Out) -> Data Type Conversion2/1
  VDDM_LimpHomeAct_flg_ovrd/1(Signal_Out) -> Data Type Conversion176/1
  VINP_BrkSwV_flg/1 -> Data Type Conversion187/1
  Data Type Conversion8/1 -> Bus Creator/9  "VINP_BrkSwSta_flg"
  Data Type Conversion187/1 -> Bus Creator/10  "VINP_BrkSwV_flg"
  ShifterHandleCmd/1(Out_signal) -> Data Type Conversion52/1
  VINP_ShifterHandleCmd_enum/1 -> ShifterHandleCmd/1(Inp_signal)
  BInInvalid_outputs/1 -> [BInInvalid_outputs]
  [BInInvalid_outputs] -> Bus Selector1/1
  Bus Selector1/1 -> ShifterHandleCmd/2(Invalid_condition)  "<VTQD_ShifterHandleCmdInV_flg>"
  ShifterFailsta/1(Out_signal) -> Data Type Conversion62/1
  VINP_ShifterFailsta_enum/1 -> ShifterFailsta/1(Inp_signal)
  [BInInvalid_outputs] -> Bus Selector2/1
  Bus Selector2/1 -> ShifterFailsta/2(Invalid_condition)  "<VTQD_ShifterFailstaInV_flg>"
  BrkSwSta/1(Out_signal) -> Data Type Conversion8/1
  VINP_BrkSwSta_flg/1 -> BrkSwSta/1(Inp_signal)
  [BInInvalid_outputs] -> Bus Selector3/1
  Bus Selector3/1 -> BrkSwSta/2(Invalid_condition)  "<VINP_BrkSwStaSWInV_flg>"
  BrkPedalPos/1(Out_signal) -> Data Type Conversion9/1
  VINP_BrkPedalPos_pct/1 -> Data Type Conversion191/1, BrkPedalPos/1(Inp_signal)
  [BInInvalid_outputs] -> Bus Selector4/1
  Bus Selector4/1 -> BrkPedalPos/2(Invalid_condition)  "<VINP_BrkPedalPosStaInV_flg>"
  Data Type Conversion191/1 -> Bus Creator/11  "VINP_BrkPedalPos_pct"
  VVMC_CCPedalOvrd_flg/1 -> Data Type Conversion7/1
  Data Type Conversion7/1 -> Bus Creator/153  "VVMC_CCPedalOvrd_flg"
  VVMC_MSAWhlTqActive_flg/1 -> Data Type Conversion188/1
  Data Type Conversion188/1 -> Bus Creator/154  "VVMC_MSAWhlTqActive_flg"
  VINP_ACCVehHoldReq_flg/1 -> Data Type Conversion189/1
  Data Type Conversion189/1 -> Bus Creator/171  "VINP_ACCVehHoldReq_flg"
  VINP_DIDExhibitMode_enum/1 -> Data Type Conversion197/1
  VINP_DIDGetDynoMode_flg/1 -> Data Type Conversion190/1
  Data Type Conversion190/1 -> Bus Creator/195  "VINP_DIDGetDynoMode_flg"
  VINP_CAN1BusOff_flg/1 -> Data Type Conversion192/1
  Data Type Conversion192/1 -> Bus Creator/196  "VINP_CAN1BusOff_flg"
  VINP_CAN1BusError_flg/1 -> Data Type Conversion193/1
  Data Type Conversion193/1 -> Bus Creator/197  "VINP_CAN1BusError_flg"
  VINP_CAN2BusOff_flg/1 -> Data Type Conversion194/1
  Data Type Conversion194/1 -> Bus Creator/198  "VINP_CAN2BusOff_flg"
  VINP_CAN2BusError_flg/1 -> Data Type Conversion195/1
  Data Type Conversion195/1 -> Bus Creator/199  "VINP_CAN2BusError_flg"
  Data Type Conversion196/1 -> Bus Creator/200  "VINP_DIDNVHPedalLim_flg"
  VINP_DIDNVHPedalLim_flg/1 -> Data Type Conversion196/1
  Data Type Conversion197/1 -> Bus Creator/194  "VINP_DIDGetExhibitMode_enum"
  VINP_SCPSystemMode_enum/1 -> Data Type Conversion198/1
  Data Type Conversion198/1 -> Bus Creator/201  "VINP_SCPSystemMode_enum"
  VDDM_EPB1NoComCFS_flg/1 -> Data Type Conversion199/1
  VDDM_EPB1RCErrCFS_flg/1 -> Data Type Conversion200/1
  VDDM_EPB1CSErrCFS_flg/1 -> Data Type Conversion201/1
  Data Type Conversion199/1 -> Bus Creator/202  "VDDM_EPB1NoComCFS_flg"
  Data Type Conversion200/1 -> Bus Creator/203  "VDDM_EPB1RCErrCFS_flg"
  Data Type Conversion201/1 -> Bus Creator/204  "VDDM_EPB1CSErrCFS_flg"
  VPMM_DrSeatSta_enum/1 -> Data Type Conversion202/1
  Data Type Conversion202/1 -> Bus Creator/7  "VPMM_DrSeatSta_enum"
  VINP_MCPressure_bar/1 -> Data Type Conversion203/1
  Data Type Conversion203/1 -> Bus Creator/45  "VINP_MCPressure_bar"
  VBCM_CTDCtrl_enum/1 -> Data Type Conversion204/1
  Data Type Conversion204/1 -> Bus Creator/205  "VBCM_CTDCtrl_enum"
  VINP_FlashCrashDetd_flg/1 -> Data Type Conversion205/1
  Data Type Conversion205/1 -> Bus Creator/206  "VINP_FlashCrashDetd_flg"
  VINP_FlashCrashUnlockReq_flg/1 -> Data Type Conversion206/1
  Data Type Conversion206/1 -> Bus Creator/207  "VINP_FlashCrashUnlockReq_flg"
  VBCM_CrashUnlkSuccess_flg/1 -> Data Type Conversion207/1
  Data Type Conversion207/1 -> Bus Creator/208  "VBCM_CrashUnlkSuccess_flg"

== system tqdtqr_rebuild_V3/SCP_In/Invalid Condition ==
  note: Shifter1 message(DDM)
  VINP_BrkSwV_flg : Inport
  VINP_BrkPedalPosSta_flg : Inport  Port=2
  VINP_ShifterHandleCmd_enum : Inport  Port=3
  VDDM_Shifter1Err_flg : Inport  Port=4
  Bus Creator : BusCreator  Inputs=4
  Constant25 : Constant  Value=KTQD_ShifterInvalidSW_flg  OutDataTypeStr=single
  Constant26 : Constant  Value=0xFF  OutDataTypeStr=single
  Constant28 : Constant  Value=KTQD_ShifterInvalidSW_flg  OutDataTypeStr=single
  Data Type Conversion : DataTypeConversion  OutDataTypeStr=boolean
  Equal8 : RelationalOperator  OutDataTypeStr=boolean  RndMeth=Simplest
  Logical Operator16 : Logic  Operator=OR  AllPortsSameDT=off  OutDataTypeStr=boolean
  Logical Operator17 : Logic  AllPortsSameDT=off  OutDataTypeStr=boolean
  Logical Operator19 : Logic  AllPortsSameDT=off  OutDataTypeStr=boolean
  Logical Operator6 : Logic  Operator=NOT  AllPortsSameDT=off  OutDataTypeStr=boolean
  BInInvalid_outputs : Outport
  wires:
  VINP_BrkSwV_flg/1 -> [VINP_BrkSwV_flg]
  [VINP_BrkSwV_flg] -> Logical Operator6/1
  VINP_BrkPedalPosSta_flg/1 -> [VINP_BrkPedalPosSta_flg]
  Data Type Conversion/1 -> [VINP_BrkPedalPosStaInV_flg]  "VINP_BrkPedalPosStaInV_flg"
  VINP_ShifterHandleCmd_enum/1 -> [VINP_ShifterHandleCmd_enum]
  VDDM_Shifter1Err_flg/1 -> [VDDM_Shifter1Err_flg]
  Constant25/1 -> Logical Operator17/2
  Equal8/1 -> Logical Operator16/2
  [VINP_ShifterHandleCmd_enum] -> Equal8/1
  [VDDM_Shifter1Err_flg] -> Logical Operator16/1
  Logical Operator16/1 -> Logical Operator17/1
  Constant26/1 -> Equal8/2
  Logical Operator17/1 -> [VTQD_ShifterHandleCmdInV_flg]  "VTQD_ShifterHandleCmdInV_flg"
  Constant28/1 -> Logical Operator19/2
  [VDDM_Shifter1Err_flg] -> Logical Operator19/1
  [VTQD_ShifterHandleCmdInV_flg] -> Bus Creator/3
  Bus Creator/1 -> BInInvalid_outputs/1  "BInInvalid_outputs"
  Logical Operator19/1 -> [VTQD_ShifterFailstaInV_flg]  "VTQD_ShifterFailstaInV_flg"
  [VTQD_ShifterFailstaInV_flg] -> Bus Creator/4
  Logical Operator6/1 -> [VINP_BrkSwStaSWInV_flg]  "VINP_BrkSwStaSWInV_flg"
  [VINP_BrkSwStaSWInV_flg] -> Bus Creator/1
  [VINP_BrkPedalPosSta_flg] -> Data Type Conversion/1
  [VINP_BrkPedalPosStaInV_flg] -> Bus Creator/2

== system tqdtqr_rebuild_V3/Input_Convert/Input Signal Convert/AWDMCUReadyExt_flg ==
  VINP_FrMCUErr_enum : Inport
  VINP_RrMCUErr_enum : Inport  Port=2
  Action Port : ActionPort  ActionPortLabel=if(u1 ~= 0)
  Constant : Constant  Value=ENUM_MCUWARN_LV0
  Constant1 : Constant  Value=ENUM_MCUWARN_NOERROR
  Constant2 : Constant  Value=ENUM_MCUWARN_LV0
  Constant3 : Constant  Value=ENUM_MCUWARN_NOERROR
  Equal{,1..3} (4 alike) : RelationalOperator  Operator===  OutDataTypeStr=boolean  RndMeth=Simplest
  Logical Operator : Logic  Operator=OR  AllPortsSameDT=off  OutDataTypeStr=boolean
  Logical Operator1 : Logic  Operator=OR  AllPortsSameDT=off  OutDataTypeStr=boolean
  Logical Operator2 : Logic  AllPortsSameDT=off  OutDataTypeStr=boolean
  VTQD_AWDMCUReadyExt_flg : Outport
  wires:
  Logical Operator1/1 -> Logical Operator2/2
  Logical Operator/1 -> Logical Operator2/1
  Constant2/1 -> Equal2/2
  VINP_RrMCUErr_enum/1 -> Equal2/1, Equal3/1
  Constant3/1 -> Equal3/2
  Equal2/1 -> Logical Operator1/1
  Equal3/1 -> Logical Operator1/2
  Constant/1 -> Equal/2
  VINP_FrMCUErr_enum/1 -> Equal/1, Equal1/1
  Constant1/1 -> Equal1/2
  Equal/1 -> Logical Operator/1
  Equal1/1 -> Logical Operator/2
  Logical Operator2/1 -> VTQD_AWDMCUReadyExt_flg/1

== system tqdtqr_rebuild_V3/Input_Convert/Input Signal Convert/FWDMCUReadyExt_flg ==
  VINP_FrMCUErr_enum : Inport
  Action Port : ActionPort  ActionPortLabel=elseif(u2 ~= 0)
  Constant : Constant  Value=ENUM_MCUWARN_LV0
  Constant1 : Constant  Value=ENUM_MCUWARN_NOERROR
  Equal : RelationalOperator  Operator===  OutDataTypeStr=boolean  RndMeth=Simplest
  Equal1 : RelationalOperator  Operator===  OutDataTypeStr=boolean  RndMeth=Simplest
  Logical Operator : Logic  Operator=OR  AllPortsSameDT=off  OutDataTypeStr=boolean
  VTQD_FWDMCUReadyExt_flg : Outport
  wires:
  Equal1/1 -> Logical Operator/2
  Constant1/1 -> Equal1/2
  Constant/1 -> Equal/2
  VINP_FrMCUErr_enum/1 -> Equal/1, Equal1/1
  Equal/1 -> Logical Operator/1
  Logical Operator/1 -> VTQD_FWDMCUReadyExt_flg/1

== system tqdtqr_rebuild_V3/Input_Convert/Input Signal Convert/RWDMCUReadyExt_flg ==
  VINP_RrMCUErr_enum : Inport
  Action Port : ActionPort  ActionPortLabel=else
  Constant : Constant  Value=ENUM_MCUWARN_LV0
  Constant1 : Constant  Value=ENUM_MCUWARN_NOERROR
  Equal : RelationalOperator  Operator===  OutDataTypeStr=boolean  RndMeth=Simplest
  Equal1 : RelationalOperator  Operator===  OutDataTypeStr=boolean  RndMeth=Simplest
  Logical Operator : Logic  Operator=OR  AllPortsSameDT=off  OutDataTypeStr=boolean
  VTQD_RWDMCUReadyExt_flg : Outport
  wires:
  Constant/1 -> Equal/2
  Constant1/1 -> Equal1/2
  Equal/1 -> Logical Operator/1
  Equal1/1 -> Logical Operator/2
  VINP_RrMCUErr_enum/1 -> Equal/1, Equal1/1
  Logical Operator/1 -> VTQD_RWDMCUReadyExt_flg/1
